simulink model "Ereg_sims_new"  (R2021b)
settings: Solver=VariableStepAuto  StartTime=0.0  StopTime=10.0  MinStep=1e-6  RelTol=1e-3
model workspace (MAT data in the model file):
  yes = 0
undefined symbols (not defined in the file): a, b, c
libraries: simulink x1, hdlsllib x1, slpidlib x1
settings Model: Creator=dymo4  LastModifiedBy=dymo4
settings OptimizationCC: BlockReduction=off  DefaultParameterBehavior=Inlined  BufferReuse=off

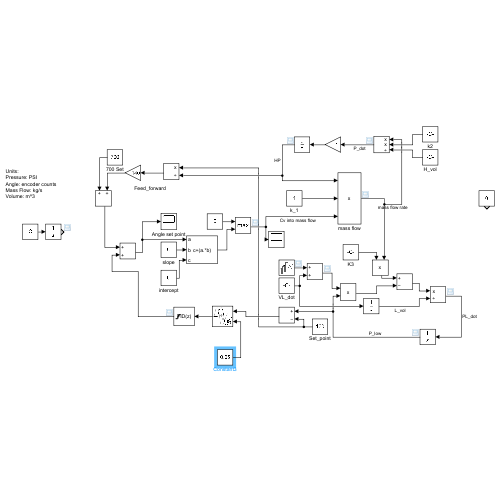
[thumbnail: Simulink's stored preview of the top-level diagram]
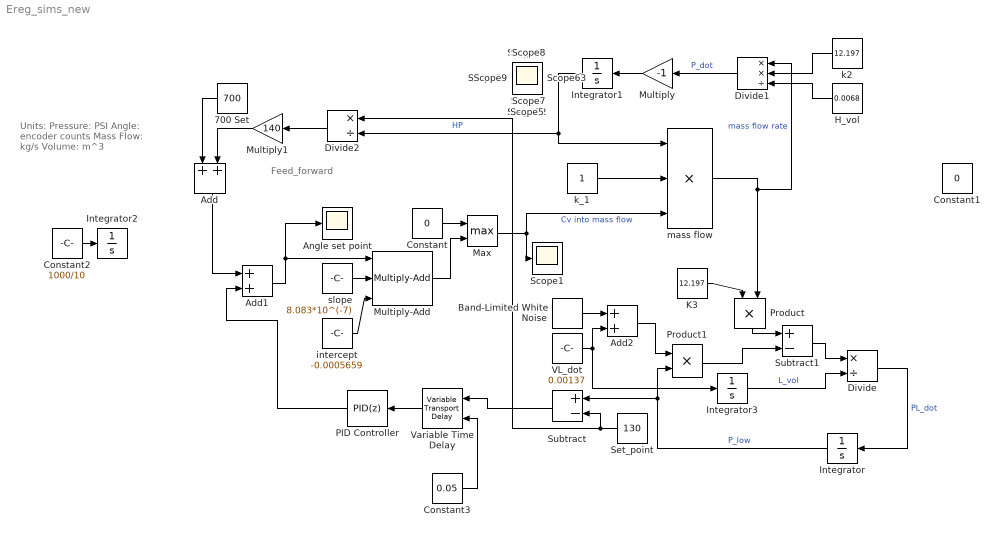
== system Ereg_sims_new ==
  note: Feed_forward
  note: Units:
      | Pressure: PSI
      | Angle: encoder counts
      | Mass Flow: kg/s
      | Volume: m^3
  700 Set : Constant  Value=700
  Add : Sum
  Add1 : Sum
  Add2 : Sum
  Angle set point : Scope
  Band-Limited White Noise : simulink/Sources/Band-Limited White Noise  Cov=[0.000000001]  Ts=.01  seed=[2331]
  Constant : Constant  Value=0
  Constant1 : Constant  Value=0
  Constant2 : Constant  Value=1000/10
  Constant3 : Constant  Value=0.05
  Divide : Product  Inputs=*/
  Divide1 : Product  Inputs=**/
  Divide2 : Product  Inputs=*/
  H_vol : Constant  Value=0.0068
  Integrator : Integrator
  Integrator1 : Integrator  InitialCondition=950
  Integrator2 : Integrator
  Integrator3 : Integrator  InitialCondition=1e-6
  K3 : Constant  Value=12.197
  Max : MinMax  Function=max  Inputs=2
  Multiply : Gain  Gain=-1
  Multiply-Add : hdlsllib/HDL Operations/Multiply-Add  Function=c+(a.*b)  datatype=Inherit: Inherit via internal rule  DoSatur=off  FMA=off
      settings: SourceProductBaseCode=SL
  Multiply1 : Gain  Gain=140
  PID Controller : slpidlib/PID Controller  Controller=PID  Form=Parallel  TimeDomain=Discrete-time  UseExternalTs=off  SampleTime=1e-3  IntegratorMethod=Forward Euler  FilterMethod=Forward Euler  ControllerParametersSource=internal  P=-6.0  I=-5  D=-1.2  UseFilter=on  N=0  TunerSelectOption=Transfer Function Based (PID Tuner App)  InitialConditionSource=internal  InitialConditionForIntegrator=0  InitialConditionForFilter=0  DifferentiatorICPrevScaledInput=0  ExternalReset=none  TrackingMode=off  Kt=1  LimitOutput=on  SatLimitsSource=internal  UpperSaturationLimit=500  LowerSaturationLimit=-500  LinearizeAsGain=on  AntiWindupMode=none  Kb=1  POutMin=[]  POutMax=[]  IOutMin=[]  IOutMax=[]  DOutMin=[]  DOutMax=[]  NOutMin=[]  NOutMax=[]  SumOutMin=[]  SumOutMax=[]  SaturationOutMin=[]  SaturationOutMax=[]  PParamMin=[]  PParamMax=[]  IParamMin=[]  IParamMax=[]  DParamMin=[]  DParamMax=[]  NParamMin=[]  NParamMax=[]  KbParamMin=[]  KbParamMax=[]  KtParamMin=[]  KtParamMax=[]  KbOutMin=[]  KbOutMax=[]  KtOutMin=[]  KtOutMax=[]  IntegratorOutMin=[]  IntegratorOutMax=[]  FilterOutMin=[]  FilterOutMax=[]  SumI1OutMin=[]  SumI1OutMax=[]  SumI2OutMin=[]  SumI2OutMax=[]  SumI3OutMin=[]  SumI3OutMax=[]  SumI4OutMin=[]  SumI4OutMax=[]  SumDOutMin=[]  SumDOutMax=[]  DifferentiatorOutMin=[]  DifferentiatorOutMax=[]  FilterDiffOutCoefMin=[]  FilterDiffOutCoefMax=[]  ReciprocalOutMin=[]  ReciprocalOutMax=[]  SumDenOutMin=[]  SumDenOutMax=[]  SumNumOutMin=[]  SumNumOutMax=[]  DivideOutMin=[]  DivideOutMax=[]  UdiffTsProdOutMin=[]  UdiffTsProdOutMax=[]  NTsProdOutMin=[]  NTsProdOutMax=[]  UintegralTsProdOutMin=[]  UintegralTsProdOutMax=[]  UngainTsProdOutMin=[]  UngainTsProdOutMax=[]  IntegratorContinuousStateAttributes=''  IntegratorStateMustResolveToSignalObject=off  IntegratorRTWStateStorageClass=Auto  FilterContinuousStateAttributes=''  FilterStateMustResolveToSignalObject=off  FilterRTWStateStorageClass=Auto  ParallelPVariant=InternalParameters  IdealPVariant=Disabled  IVariant=InternalParameters  DVariant=InternalParameters  IntegratorVariant=Discrete  SatVariant=Enabled  AWVariant=Passthrough  PCopyVariant=Disabled  TRVariant=Disabled  FdbkBlocksVariant=Forward  IdealPFdbkVariant=Disabled  SatFdbkVariant=Disabled  DerivativeFilterVariant=ForwardEulerFilter  NVariant=InternalParameters  NCopyVariant=Disabled  FilterICVariant=InternalICsFilter  IntegratorICVariant=InternalICs  ExternalResetVariant=Disabled  TRSumVariant=Passthrough  SumFdbkVariant=Disabled  SumVariant=Sum_PID  TsampFilterVariant=InternalTs  TsampNgainVariant=Passthrough  TsampIntegralVariant=Passthrough  ExternalSaturationOutDataTypeStr=Inherit: Same as second input
  Product : Product
  Product1 : Product
  Scope{,1..13} (14 alike) : Scope
  Set_point : Constant  Value=130
  Subtract : Sum  Inputs=+-
  Subtract1 : Sum  Inputs=+-
  VL_dot : Constant  Value=0.00137
  Variable Time Delay : VariableTransportDelay  MaximumDelay=10
  intercept : Constant  Value=-0.0005659
  k2 : Constant  Value=12.197
  k_1 : Constant
  mass flow : Product  Inputs=3
  slope : Constant  Value=8.083*10^(-7)
  wires:
  k_1/1 -> mass flow/2
  Constant/1 -> Max/1
  slope/1 -> Multiply-Add/2
  intercept/1 -> Multiply-Add/3
  Multiply-Add/1 -> Max/2
  Max/1 -> mass flow/3, Scope1/1  "Cv into mass flow"
  PID Controller/1 -> Add1/2
  mass flow/1 -> Product/2, Divide1/1  "mass flow rate"
  Integrator3/1 -> Divide/2  "L_vol"
  K3/1 -> Product/1
  Product/1 -> Subtract1/1
  Integrator/1 -> Product1/2, Subtract/1  "P_low"
  VL_dot/1 -> Integrator3/1, Add2/2
  Product1/1 -> Subtract1/2
  Subtract1/1 -> Divide/1
  Divide/1 -> Integrator/1  "PL_dot"
  k2/1 -> Divide1/2
  H_vol/1 -> Divide1/3
  Divide1/1 -> Multiply/1  "P_dot"
  Integrator1/1 -> Divide2/2, mass flow/1  "HP"
  Multiply/1 -> Integrator1/1
  Set_point/1 -> Divide2/1, Subtract/2
  Constant2/1 -> Integrator2/1
  700 Set/1 -> Add/1
  Divide2/1 -> Multiply1/1
  Multiply1/1 -> Add/2
  Add1/1 -> Multiply-Add/1, Angle set point/1
  Add/1 -> Add1/1
  Band-Limited White Noise/1 -> Add2/1
  Add2/1 -> Product1/1
  Variable Time Delay/1 -> PID Controller/1
  Constant3/1 -> Variable Time Delay/2
  Subtract/1 -> Variable Time Delay/1
